simulink model "q_hfe_open_loop"  (Simulink 7.4)
settings: Solver=FixedStepDiscrete  StartTime=0.0  StopTime=inf  FixedStep=0.01  RelTol=1e-3
values from neighbouring files (symbols this model uses):
  K_TACH = K_TACH_V2HZ * HZ2RPM    (= 1063.8)    [setup_hfe.m]
  K_TEMP = 20    [setup_hfe.m]
undefined symbols (not defined in the file or in its folder): Heatflow, hfe_lib, HIL, qc_get_step_size
libraries: quarc_library x5, simulink x1
settings Model: Creator=MLevis  LastModifiedBy=EE406  SimulationMode=external  ExtModeTrigDuration=30000
settings SolverCC: PositivePriorityOrder=on
settings OptimizationCC: InitFltsAndDblsToZero=on
settings DebuggingCC: SaveWithParameterizedLinksMsg=none
settings RTWCC: SystemTargetFile=quarc_windows.tlc  TemplateMakefile=quarc_default_tmf  Description=QUARC Win32 Target  ProcessScript=quarc_windows_make_rtw_hook
settings STFCustomTargetCC: TargetPreCompLibLocation=C:\DOCUME~1\ALLUSE~1\APPLIC~1\QUARC\lib\2009b\windows\release  GeneratePreprocessorConditionals=Disable all  SystemTargetFile=quarc_windows.tlc
settings GRTTargetCC: TargetPreCompLibLocation=C:\DOCUME~1\ALLUSE~1\APPLIC~1\QUARC\lib\2009b\windows\release  ParMdlRefBuildCompliant=off  CompOptLevelCompliant=off  MatFileLogging=off  ExtMode=on  ExtModeMexFile=quarc_comm

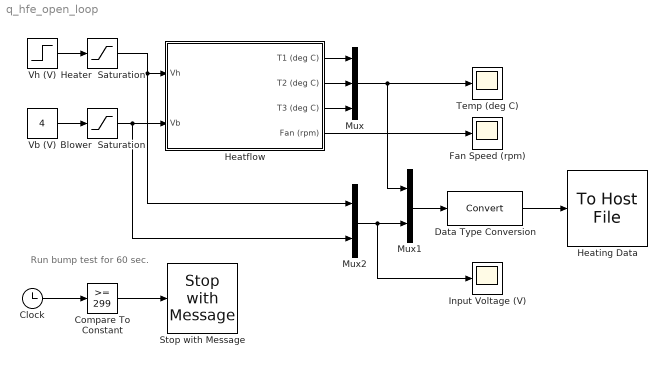
== system q_hfe_open_loop ==
  note: Run bump test for 60 sec.
  Blower  Saturation : Saturate  UpperLimit=6  LowerLimit=0
  Clock : Clock
      settings: Decimation=10
  Compare To Constant : simulink/Logic and Bit Operations/Compare To Constant  SystemSampleTime=-1  relop=>=  const=299  LogicOutDataTypeMode=uint8
  Data Type Conversion : DataTypeConversion
  Fan Speed (rpm) : Scope
      settings: TimeRange=300  YMin=1000  YMax=2000  SaveName=data_spd  DataFormat=Array  MaxDataPoints=6000
  Heater  Saturation : Saturate  UpperLimit=5  LowerLimit=0
  Heatflow : Subsystem  AncestorBlock=hfe_lib/Heatflow
  Heating Data : quarc_library/Sinks/To Host/To Host File  file_name=data_open_loop.mat  variable_name=data_hfe_ol  decimation=1  sample_time=qc_get_step_size  file_format=MAT-file v.4  options=No header or footer  append=off  final_file_name=data_open_loop.mat
      settings: AttributesFormatString=%<file_name>
  Input Voltage (V) : Scope
      settings: TimeRange=300  YMin=-1  YMax=6  SaveName=data_spd1  DataFormat=Array  MaxDataPoints=6000
  Mux : Mux  Inputs=3
  Mux1 : Mux  Inputs=2
  Mux2 : Mux  Inputs=2
  Stop with Message : quarc_library/Sinks/Error Handling/Stop with Message  SystemSampleTime=-1  message_type=Fixed error message  message_icon=Information  message=Bump test complete.
  Temp (deg C) : Scope
      settings: TimeRange=300  YMin=30  YMax=105  SaveName=data_temp  DataFormat=Array  MaxDataPoints=6000
  Vb (V) : Constant  Value=4
  Vh (V) : Step  Time=5  After=4  SampleTime=0
  wires:
  Vb (V)/1 -> Blower  Saturation/1
  Vh (V)/1 -> Heater  Saturation/1
  Heatflow/4(Fan (rpm)) -> Fan Speed (rpm)/1
  Heatflow/1(T1 (deg C)) -> Mux/1
  Heatflow/2(T2 (deg C)) -> Mux/2
  Heatflow/3(T3 (deg C)) -> Mux/3
  Mux/1 -> Temp (deg C)/1, Mux1/1
  Mux1/1 -> Data Type Conversion/1
  Data Type Conversion/1 -> Heating Data/1
  Mux2/1 -> Mux1/2, Input Voltage (V)/1
  Heater  Saturation/1 -> Heatflow/1(Vh), Mux2/1
  Blower  Saturation/1 -> Heatflow/2(Vb), Mux2/2
  Clock/1 -> Compare To Constant/1
  Compare To Constant/1 -> Stop with Message/1

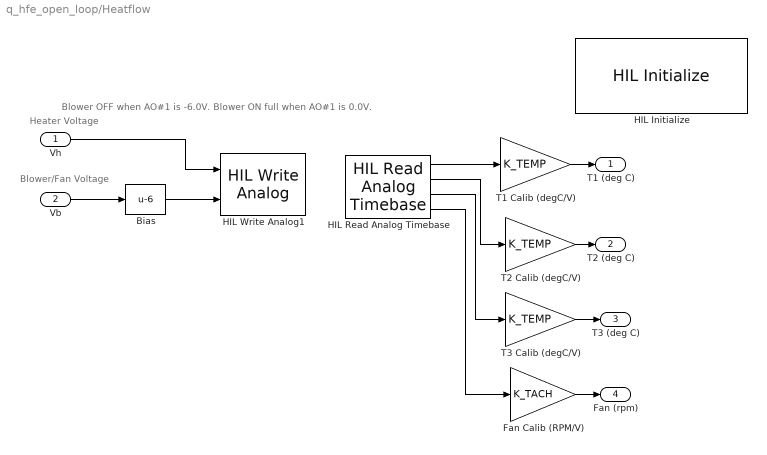
== system q_hfe_open_loop/Heatflow ==
  note: Heater Voltage
  note: Blower/Fan Voltage
  note: Blower OFF when AO#1 is -6.0V.
      | Blower ON full when AO#1 is 0.0V.
  Vh : Inport
  Vb : Inport  Port=2
  Bias : Bias  Bias=-6
  Fan Calib (RPM/V) : Gain  Gain=K_TACH
  HIL Initialize : quarc_library/Data Acquisition/Generic/Configuration/HIL Initialize  object_name=HIL-1  board_type=q8_usb  board_number=0  board_options=update_rate=normal  exclusive=off  active=on  hardware_clocks=[0:2]  clock_modes=[]  set_clock_params_at_start=off  set_clock_params_at_switch_in=off  analog_input_channels=[0:7]  analog_input_maximums=10  analog_input_minimums=-10  set_analog_input_params_at_start=on  set_analog_input_params_at_switch_in=off  analog_output_channels=[0:7]  analog_output_maximums=10  analog_output_minimums=-10  initial_analog_outputs=[0]  final_analog_outputs=[0]  watchdog_analog_outputs=0  set_analog_output_params_at_start=on  set_analog_output_params_at_switch_in=off  set_analog_outputs_at_start=on  set_analog_outputs_at_switch_in=off  set_analog_outputs_at_terminate=on  set_analog_outputs_at_switch_out=off  set_analog_outputs_on_watchdog=off  digital_input_channels=[]  digital_output_channels=[]  digital_output_configuration=[]  initial_digital_outputs=[1]  final_digital_outputs=[1]  watchdog_digital_outputs=[1]  set_digital_output_params_at_start=off  set_digital_output_params_at_switch_in=off  set_digital_outputs_at_start=on  set_digital_outputs_at_switch_in=off  set_digital_outputs_at_terminate=on  set_digital_outputs_at_switch_out=off  set_digital_outputs_on_watchdog=off  encoder_channels=[0:7]  quadrature=[4]  encoder_filter_frequency=[]  initial_encoder_counts=[0]  set_encoder_params_at_start=on  set_encoder_params_at_switch_in=off  set_encoder_counts_at_start=on  set_encoder_counts_at_switch_in=off  pwm_channels=[0:7]  pwm_modes=0  pwm_frequency=99.532799999999995e6/4095  pwm_configuration=[0]  pwm_alignment=[0]  pwm_polarity=[1]  pwm_leading_deadband=[0]  pwm_trailing_deadband=[0]  initial_pwm_outputs=[0]  final_pwm_outputs=[0]  watchdog_pwm_outputs=[0]  set_pwm_params_at_start=on  set_pwm_params_at_switch_in=off  set_pwm_outputs_at_start=on  set_pwm_outputs_at_switch_in=off  set_pwm_outputs_at_terminate=on  set_pwm_outputs_at_switch_out=off  set_pwm_outputs_on_watchdog=off  other_output_channels=[]  initial_other_outputs=[]  final_other_outputs=[]  watchdog_other_outputs=[]  set_other_outputs_at_start=off  set_other_outputs_at_switch_in=off  set_other_outputs_at_terminate=off  set_other_outputs_at_switch_out=off  set_other_outputs_on_watchdog=off
  HIL Read Analog Timebase : quarc_library/Data Acquisition/Generic/Timebases/HIL Read Analog Timebase  object_name=HIL-1  clock=0  channels=[0:3]  samples_in_buffer=max(ceil(1/qc_get_step_size), 1)  active=on  vector_output=off
      settings: AttributesFormatString=(%<object_name>)
  HIL Write Analog1 : quarc_library/Data Acquisition/Generic/Immediate I//O/HIL Write Analog  object_name=HIL-1  channels=[0,1]  sample_time=-1  active=off  vector_input=off
  T1 Calib (degC/V) : Gain  Gain=K_TEMP
  T2 Calib (degC/V) : Gain  Gain=K_TEMP
  T3 Calib (degC/V) : Gain  Gain=K_TEMP
  T1 (deg C) : Outport
  T2 (deg C) : Outport  Port=2
  T3 (deg C) : Outport  Port=3
  Fan (rpm) : Outport  Port=4
  wires:
  T3 Calib (degC/V)/1 -> T3 (deg C)/1
  T2 Calib (degC/V)/1 -> T2 (deg C)/1
  Vh/1 -> HIL Write Analog1/1
  HIL Read Analog Timebase/4 -> Fan Calib (RPM/V)/1
  Vb/1 -> Bias/1
  HIL Read Analog Timebase/3 -> T3 Calib (degC/V)/1
  HIL Read Analog Timebase/2 -> T2 Calib (degC/V)/1
  HIL Read Analog Timebase/1 -> T1 Calib (degC/V)/1
  T1 Calib (degC/V)/1 -> T1 (deg C)/1
  Fan Calib (RPM/V)/1 -> Fan (rpm)/1
  Bias/1 -> HIL Write Analog1/2
